simulink model "D53_LKAS_JLU_20200909_1512"  (R2018b)
settings: Solver=ode3  StartTime=0.0  StopTime=10.0  FixedStep=0.01  RelTol=1e-3  EnableMultiTasking=on
model workspace (MAT data in the model file):
  MCOS : class17 (value not decoded)
  MCOS : class17 (value not decoded)
  MCOS : class17 (value not decoded)
  MCOS : class17 (value not decoded)
  MCOS : class17 (value not decoded)
  MCOS : class17 (value not decoded)
  MCOS : class17 (value not decoded)
  MCOS : class17 (value not decoded)
  MCOS : class17 (value not decoded)
  MCOS : class17 (value not decoded)
  MCOS : class17 (value not decoded)
  MCOS : class17 (value not decoded)
  MCOS : class17 (value not decoded)
  MCOS : class17 (value not decoded)
  MCOS : class17 (value not decoded)
  MCOS : class17 (value not decoded)
  MCOS : class17 (value not decoded)
  MCOS : class17 (value not decoded)
  MCOS : class17 (value not decoded)
  MCOS : class17 (value not decoded)
  MCOS : class17 (value not decoded)
  MCOS : class17 (value not decoded)
  MCOS : class17 (value not decoded)
  MCOS : class17 (value not decoded)
  MCOS : class17 (value not decoded)
  MCOS : class17 (value not decoded)
  MCOS : class17 (value not decoded)
  MCOS : class17 (value not decoded)
  MCOS : class17 (value not decoded)
  MCOS : class17 (value not decoded)
  MCOS : class17 (value not decoded)
  MCOS : class17 (value not decoded)
  MCOS : class17 (value not decoded)
  MCOS : class17 (value not decoded)
  MCOS : class17 (value not decoded)
  MCOS : class17 (value not decoded)
  MCOS : class17 (value not decoded)
  MCOS : class17 (value not decoded)
  MCOS : class17 (value not decoded)
  MCOS : class17 (value not decoded)
  MCOS : class17 (value not decoded)
  MCOS : class17 (value not decoded)
  MCOS : class17 (value not decoded)
  MCOS : class17 (value not decoded)
  MCOS : class17 (value not decoded)
  MCOS : class17 (value not decoded)
  MCOS : class17 (value not decoded)
  MCOS : class17 (value not decoded)
  MCOS : class17 (value not decoded)
  MCOS : class17 (value not decoded)
  MCOS : class17 (value not decoded)
  MCOS : class17 (value not decoded)
  MCOS : class17 (value not decoded)
  MCOS : class17 (value not decoded)
  MCOS : class17 (value not decoded)
  MCOS : class17 (value not decoded)
  MCOS : class17 (value not decoded)
  MCOS : class17 (value not decoded)
  MCOS : class17 (value not decoded)
  MCOS : class17 (value not decoded)
  MCOS : class17 (value not decoded)
  MCOS : class17 (value not decoded)
  MCOS : class17 (value not decoded)
  MCOS : class17 (value not decoded)
  MCOS : class17 (value not decoded)
  MCOS : class17 (value not decoded)
  MCOS : class17 (value not decoded)
  MCOS : class17 (value not decoded)
  MCOS : class17 (value not decoded)
  MCOS : class17 (value not decoded)
  MCOS : class17 (value not decoded)
  MCOS : class17 (value not decoded)
  MCOS : class17 (value not decoded)
  MCOS : class17 (value not decoded)
  MCOS : class17 (value not decoded)
  MCOS : class17 (value not decoded)
  MCOS : class17 (value not decoded)
  MCOS : class17 (value not decoded)
  MCOS : class17 (value not decoded)
  MCOS : class17 (value not decoded)
  MCOS : class17 (value not decoded)
  MCOS : class17 (value not decoded)
  MCOS : class17 (value not decoded)
  MCOS : class17 (value not decoded)
  MCOS : class17 (value not decoded)
  MCOS : class17 (value not decoded)
  MCOS : class17 (value not decoded)
  MCOS : class17 (value not decoded)
  MCOS : class17 (value not decoded)
undefined symbols (not defined in the file): LKA_CarWidth, LKA_SampleTime, LKA_StrRatio_C, LKA_Veh2CamL_C, LKA_Veh2CamW_C, LKA_WhlBaseL_C, LL_CompSWA_C, LL_CrvtPrvwT_C, LL_DesDvt_C, LL_DvtComp_C, LL_DvtPrvwT_C, LL_DvtSpdDet_vDvtSpdMin_C, LL_HdAgExT_C, LL_HdAgPrvwT_C, LL_LAccMax_C, LL_LAccRMax_C, LL_LDW_EarliestWarnLine_C, LL_LDW_LatestWarnLine_C, LL_LDWS_SUPPRESS_HEADING, LL_LFClb_TFC_DiffCtlBalance, LL_LFClb_TFC_DiffCtrlMaxSWA, LL_LFClb_TFC_DiffCtrlRatio, LL_LFClb_TFC_facmGainLutGain1_C, LL_LFClb_TFC_facmGainLutGain2_C, LL_LFClb_TFC_facmIntegRatio, LL_LFClb_TFC_facmKlat_C, LL_LFClb_TFC_FfCtlRatio_C, LL_LFClb_TFC_phiIntegCtlMaxSWA_C, LL_LFClb_TFC_tiKlatPrvwT_C, LL_LFClb_TFC_vGainLutVehSpdLwr_C, LL_LFClb_TFC_vGainLutVehSpdUpr_C, LL_LKA_EarliestWarnLine_C, LL_LKA_LatestWarnLine_C, LL_LKAExPrcs_ExitC0Dvt, LL_LKAExPrcs_ExitC0Swt, LL_LKAExPrcs_tiExitTime1, LL_LKAExPrcs_tiExitTime2, LL_LKAExPrcs_tiExitTime3, LL_LKAS_OUT_OF_CONTROL_LAT_VEL, LL_LKAS_OUT_OF_CONTROL_TTLC, LL_LKASWASyn_M0, LL_LKASWASyn_M1, LL_LKASWASyn_M2, LL_LKASWASyn_M3K, LL_LKASWASyn_SWAaddMax, LL_LKASWASyn_T2, LL_LKASWASyn_tiTrqSwaRtTime, LL_LKASWASyn_tiTrqSwaTime, LL_LKASWASyn_TrqMax, LL_LKASWASyn_TrqSwaAddSwt, LL_LKASWASyn_TrqSwaRateDiff, LL_LSpdCompT_C, LL_lStpLngth_C, LL_MAX_DELAY_EPSSTAR_TIME, LL_MAX_DRIVER_TORQUE_DISABLE, LL_MAX_DRIVER_TORQUE_ENABLE, LL_MAX_LANE_WIDTH_DISABLE, LL_MAX_LANE_WIDTH_ENABLE, LL_MAX_LAT_ACC_DISABLE, LL_MAX_LAT_ACC_ENABLE ... (+30)
libraries: simulink x134, canmsglib x50, dspstat3 x3, simulink_extras x1
(part 4 of 17)

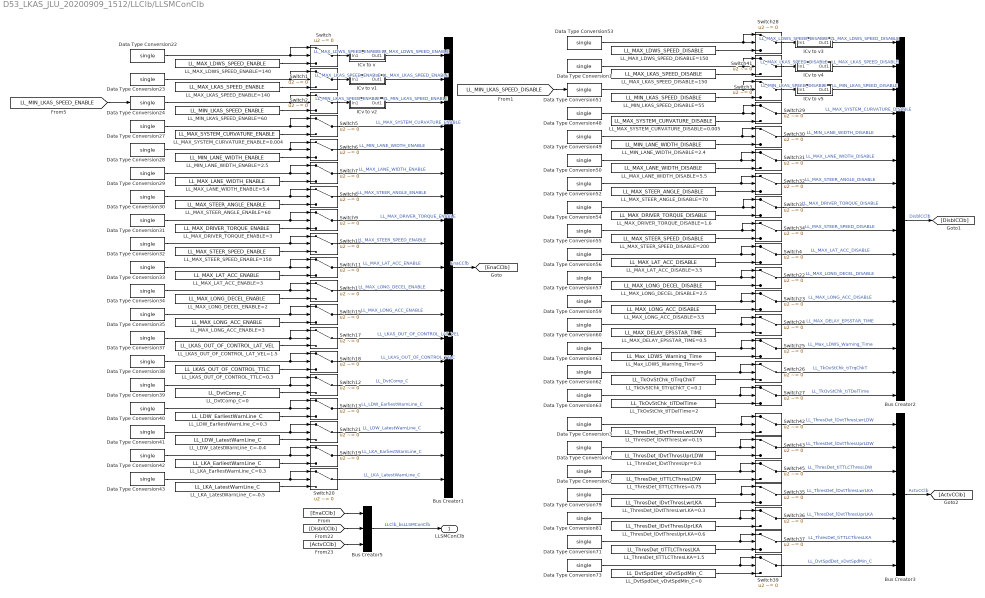
== system D53_LKAS_JLU_20200909_1512/LLClb/LLSMConClb ==
  Bus Creator1 : BusCreator  Inputs=19
  Bus Creator2 : BusCreator  Inputs=16
  Bus Creator3 : BusCreator  Inputs=7
  Bus Creator5 : BusCreator  Inputs=3
  Data Type Conversion{1..4,22..24,27..35,37..43,48..57,59..63,71,73,79,81} (42 alike) : DataTypeConversion  OutDataTypeStr=single
  ICv to v : Subsystem
  ICv to v1 : Subsystem
  ICv to v2 : Subsystem
  ICv to v3 : Subsystem
  ICv to v4 : Subsystem
  ICv to v5 : Subsystem
  LL_DvtComp_C=0 : Constant  Value=LL_DvtComp_C  OutDataTypeStr=single
  LL_DvtSpdDet_vDvtSpdMin_C=0 : Constant  Value=LL_DvtSpdDet_vDvtSpdMin_C  OutDataTypeStr=single
  LL_LDW_EarliestWarnLine_C=0.3 : Constant  Value=LL_LDW_EarliestWarnLine_C  OutDataTypeStr=single
  LL_LDW_LatestWarnLine_C=-0.4 : Constant  Value=LL_LDW_LatestWarnLine_C  OutDataTypeStr=single
  LL_LKAS_OUT_OF_CONTROL_LAT_VEL=1.5 : Constant  Value=LL_LKAS_OUT_OF_CONTROL_LAT_VEL  OutDataTypeStr=single
  LL_LKAS_OUT_OF_CONTROL_TTLC=0.3 : Constant  Value=LL_LKAS_OUT_OF_CONTROL_TTLC  OutDataTypeStr=single
  LL_LKA_EarliestWarnLine_C=0.3 : Constant  Value=LL_LKA_EarliestWarnLine_C  OutDataTypeStr=single
  LL_LKA_LatestWarnLine_C=-0.5 : Constant  Value=LL_LKA_LatestWarnLine_C  OutDataTypeStr=single
  LL_MAX_DELAY_EPSSTAR_TIME=0.5 : Constant  Value=LL_MAX_DELAY_EPSSTAR_TIME  OutDataTypeStr=single
  LL_MAX_DRIVER_TORQUE_DISABLE=1.6 : Constant  Value=LL_MAX_DRIVER_TORQUE_DISABLE  OutDataTypeStr=single
  LL_MAX_DRIVER_TORQUE_ENABLE=3 : Constant  Value=LL_MAX_DRIVER_TORQUE_ENABLE  OutDataTypeStr=single
  LL_MAX_LANE_WIDTH_DISABLE=5.5 : Constant  Value=LL_MAX_LANE_WIDTH_DISABLE  OutDataTypeStr=single
  LL_MAX_LANE_WIDTH_ENABLE=5.4 : Constant  Value=LL_MAX_LANE_WIDTH_ENABLE  OutDataTypeStr=single
  LL_MAX_LAT_ACC_DISABLE=3.5 : Constant  Value=LL_MAX_LAT_ACC_DISABLE  OutDataTypeStr=single
  LL_MAX_LAT_ACC_ENABLE=3 : Constant  Value=LL_MAX_LAT_ACC_ENABLE  OutDataTypeStr=single
  LL_MAX_LDWS_SPEED_DISABLE=150 : Constant  Value=LL_MAX_LDWS_SPEED_DISABLE  OutDataTypeStr=single
  LL_MAX_LDWS_SPEED_ENABLE=140 : Constant  Value=LL_MAX_LDWS_SPEED_ENABLE  OutDataTypeStr=single
  LL_MAX_LKAS_SPEED_DISABLE=150 : Constant  Value=LL_MAX_LKAS_SPEED_DISABLE  OutDataTypeStr=single
  LL_MAX_LKAS_SPEED_ENABLE=140 : Constant  Value=LL_MAX_LKAS_SPEED_ENABLE  OutDataTypeStr=single
  LL_MAX_LONG_ACC_DISABLE=3.5 : Constant  Value=LL_MAX_LONG_ACC_DISABLE  OutDataTypeStr=single
  LL_MAX_LONG_ACC_ENABLE=3 : Constant  Value=LL_MAX_LONG_ACC_ENABLE  OutDataTypeStr=single
  LL_MAX_LONG_DECEL_DISABLE=2.5 : Constant  Value=LL_MAX_LONG_DECEL_DISABLE  OutDataTypeStr=single
  LL_MAX_LONG_DECEL_ENABLE=2 : Constant  Value=LL_MAX_LONG_DECEL_ENABLE  OutDataTypeStr=single
  LL_MAX_STEER_ANGLE_DISABLE=70 : Constant  Value=LL_MAX_STEER_ANGLE_DISABLE  OutDataTypeStr=single
  LL_MAX_STEER_ANGLE_ENABLE=60 : Constant  Value=LL_MAX_STEER_ANGLE_ENABLE  OutDataTypeStr=single
  LL_MAX_STEER_SPEED_DISABLE=200 : Constant  Value=LL_MAX_STEER_SPEED_DISABLE  OutDataTypeStr=single
  LL_MAX_STEER_SPEED_ENABLE=150 : Constant  Value=LL_MAX_STEER_SPEED_ENABLE  OutDataTypeStr=single
  LL_MAX_SYSTEM_CURVATURE_DISABLE=0.005 : Constant  Value=LL_MAX_SYSTEM_CURVATURE_DISABLE  OutDataTypeStr=single
  LL_MAX_SYSTEM_CURVATURE_ENABLE=0.004 : Constant  Value=LL_MAX_SYSTEM_CURVATURE_ENABLE  OutDataTypeStr=single
  LL_MIN_LANE_WIDTH_DISABLE=2.4 : Constant  Value=LL_MIN_LANE_WIDTH_DISABLE  OutDataTypeStr=single
  LL_MIN_LANE_WIDTH_ENABLE=2.5 : Constant  Value=LL_MIN_LANE_WIDTH_ENABLE  OutDataTypeStr=single
  LL_MIN_LKAS_SPEED_DISABLE=55 : Constant  Value=LL_MIN_LKAS_SPEED_DISABLE  OutDataTypeStr=single
  LL_MIN_LKAS_SPEED_ENABLE=60 : Constant  Value=LL_MIN_LKAS_SPEED_ENABLE  OutDataTypeStr=single
  LL_Max_LDWS_Warning_Time=5 : Constant  Value=LL_Max_LDWS_Warning_Time  OutDataTypeStr=single
  LL_ThresDet_lDvtThresLwr=0.15 : Constant  Value=LL_ThresDet_lDvtThresLwrLDW  OutDataTypeStr=single
  LL_ThresDet_lDvtThresLwrLKA=0.3 : Constant  Value=LL_ThresDet_lDvtThresLwrLKA  OutDataTypeStr=single
  LL_ThresDet_lDvtThresUpr=0.3 : Constant  Value=LL_ThresDet_lDvtThresUprLDW  OutDataTypeStr=single
  LL_ThresDet_lDvtThresUprLKA=0.6 : Constant  Value=LL_ThresDet_lDvtThresUprLKA  OutDataTypeStr=single
  LL_ThresDet_tiTTLCThres=0.75 : Constant  Value=LL_ThresDet_tiTTLCThresLDW  OutDataTypeStr=single
  LL_ThresDet_tiTTLCThresLKA=1.5 : Constant  Value=LL_ThresDet_tiTTLCThresLKA  OutDataTypeStr=single
  LL_TkOvStChk_tiTDelTime=2 : Constant  Value=LL_TkOvStChk_tiTDelTime  OutDataTypeStr=single
  LL_TkOvStChk_tiTrqChkT_C=0.1 : Constant  Value=LL_TkOvStChk_tiTrqChkT  OutDataTypeStr=single
  Switch{,1..15,17..37,39,41..43,45} (42 alike) : Switch  Criteria=u2 ~= 0  OutDataTypeStr=single
  LLSMConClb : Outport
  wires:
  Data Type Conversion39/1 -> Switch12/2, Switch12/1
  Switch10/1 -> Bus Creator1/9  "LL_MAX_STEER_SPEED_ENABLE"
  LL_MAX_LANE_WIDTH_ENABLE=5.4/1 -> Switch7/3
  Data Type Conversion42/1 -> Switch19/2, Switch19/1
  ICv to v2/1(Out1) -> Bus Creator1/3  "LL_MIN_LKAS_SPEED_ENABLE"
  LL_LKA_LatestWarnLine_C=-0.5/1 -> Switch20/3
  Data Type Conversion40/1 -> Switch13/2, Switch13/1
  LL_MAX_STEER_ANGLE_ENABLE=60/1 -> Switch8/3
  Data Type Conversion38/1 -> Switch18/2, Switch18/1
  Data Type Conversion43/1 -> Switch20/2, Switch20/1
  LL_MIN_LANE_WIDTH_ENABLE=2.5/1 -> Switch6/3
  Switch6/1 -> Bus Creator1/5  "LL_MIN_LANE_WIDTH_ENABLE"
  Switch17/1 -> Bus Creator1/13  "LL_LKAS_OUT_OF_CONTROL_LAT_VEL"
  LL_MAX_LONG_DECEL_ENABLE=2/1 -> Switch14/3
  Data Type Conversion30/1 -> Switch8/2, Switch8/1
  Data Type Conversion27/1 -> Switch5/2, Switch5/1
  Data Type Conversion31/1 -> Switch9/2, Switch9/1
  Data Type Conversion28/1 -> Switch6/2, Switch6/1
  LL_LKAS_OUT_OF_CONTROL_LAT_VEL=1.5/1 -> Switch17/3
  Data Type Conversion23/1 -> Switch1/2, Switch1/1
  LL_MIN_LKAS_SPEED_ENABLE=60/1 -> Switch2/3
  Data Type Conversion22/1 -> Switch/2, Switch/1
  Data Type Conversion24/1 -> Switch2/2, Switch2/1
  LL_MAX_LAT_ACC_ENABLE=3/1 -> Switch11/3
  LL_MAX_LDWS_SPEED_ENABLE=140/1 -> Switch/3
  Switch12/1 -> Bus Creator1/15  "LL_DvtComp_C"
  LL_LDW_LatestWarnLine_C=-0.4/1 -> Switch21/3
  Data Type Conversion29/1 -> Switch7/2, Switch7/1
  LL_MAX_LONG_ACC_ENABLE=3/1 -> Switch15/3
  LL_MAX_DRIVER_TORQUE_ENABLE=3/1 -> Switch9/3
  Data Type Conversion35/1 -> Switch15/2, Switch15/1
  LL_DvtComp_C=0/1 -> Switch12/3
  Switch19/1 -> Bus Creator1/18  "LL_LKA_EarliestWarnLine_C"
  LL_LKAS_OUT_OF_CONTROL_TTLC=0.3/1 -> Switch18/3
  Data Type Conversion32/1 -> Switch10/2, Switch10/1
  Data Type Conversion37/1 -> Switch17/2, Switch17/1
  Data Type Conversion33/1 -> Switch11/2, Switch11/1
  Switch7/1 -> Bus Creator1/6  "LL_MAX_LANE_WIDTH_ENABLE"
  Data Type Conversion34/1 -> Switch14/2, Switch14/1
  LL_LKA_EarliestWarnLine_C=0.3/1 -> Switch19/3
  Switch15/1 -> Bus Creator1/12  "LL_MAX_LONG_ACC_ENABLE"
  Switch18/1 -> Bus Creator1/14  "LL_LKAS_OUT_OF_CONTROL_TTLC"
  Switch21/1 -> Bus Creator1/17  "LL_LDW_LatestWarnLine_C"
  ICv to v/1(Out1) -> Bus Creator1/1  "LL_MAX_LDWS_SPEED_ENABLE"
  Switch20/1 -> Bus Creator1/19  "LL_LKA_LatestWarnLine_C"
  Switch14/1 -> Bus Creator1/11  "LL_MAX_LONG_DECEL_ENABLE"
  Switch13/1 -> Bus Creator1/16  "LL_LDW_EarliestWarnLine_C"
  Switch9/1 -> Bus Creator1/8  "LL_MAX_DRIVER_TORQUE_ENABLE"
  LL_MAX_STEER_SPEED_ENABLE=150/1 -> Switch10/3
  LL_MAX_SYSTEM_CURVATURE_ENABLE=0.004/1 -> Switch5/3
  Switch5/1 -> Bus Creator1/4  "LL_MAX_SYSTEM_CURVATURE_ENABLE"
  Switch8/1 -> Bus Creator1/7  "LL_MAX_STEER_ANGLE_ENABLE"
  Data Type Conversion41/1 -> Switch21/2, Switch21/1
  LL_LDW_EarliestWarnLine_C=0.3/1 -> Switch13/3
  ICv to v1/1(Out1) -> Bus Creator1/2  "LL_MAX_LKAS_SPEED_ENABLE"
  LL_MAX_LKAS_SPEED_ENABLE=140/1 -> Switch1/3
  Switch11/1 -> Bus Creator1/10  "LL_MAX_LAT_ACC_ENABLE"
  Data Type Conversion54/1 -> Switch33/2, Switch33/1
  Data Type Conversion63/1 -> Switch27/2, Switch27/1
  Data Type Conversion52/1 -> Switch32/2, Switch32/1
  Data Type Conversion61/1 -> Switch25/2, Switch25/1
  Switch26/1 -> Bus Creator2/15  "LL_TkOvStChk_tiTrqChkT"
  LL_MIN_LKAS_SPEED_DISABLE=55/1 -> Switch3/3
  Data Type Conversion60/1 -> Switch24/2, Switch24/1
  Data Type Conversion59/1 -> Switch23/2, Switch23/1
  Data Type Conversion49/1 -> Switch30/2, Switch30/1
  Switch30/1 -> Bus Creator2/5  "LL_MIN_LANE_WIDTH_DISABLE"
  Data Type Conversion62/1 -> Switch26/2, Switch26/1
  LL_MAX_LONG_DECEL_DISABLE=2.5/1 -> Switch22/3
  Switch25/1 -> Bus Creator2/14  "LL_Max_LDWS_Warning_Time"
  Data Type Conversion57/1 -> Switch22/1, Switch22/2
  Switch29/1 -> Bus Creator2/4  "LL_MAX_SYSTEM_CURVATURE_DISABLE"
  Data Type Conversion48/1 -> Switch29/2, Switch29/1
  LL_MAX_SYSTEM_CURVATURE_DISABLE=0.005/1 -> Switch29/3
  Switch23/1 -> Bus Creator2/12  "LL_MAX_LONG_ACC_DISABLE"
  LL_MAX_DELAY_EPSSTAR_TIME=0.5/1 -> Switch24/3
  Data Type Conversion53/1 -> Switch28/2, Switch28/1
  LL_MAX_DRIVER_TORQUE_DISABLE=1.6/1 -> Switch33/3
  LL_MAX_LANE_WIDTH_DISABLE=5.5/1 -> Switch31/3
  LL_TkOvStChk_tiTrqChkT_C=0.1/1 -> Switch26/3
  LL_MAX_LDWS_SPEED_DISABLE=150/1 -> Switch28/3
  Switch4/1 -> Bus Creator2/10  "LL_MAX_LAT_ACC_DISABLE"
  Data Type Conversion50/1 -> Switch31/2, Switch31/1
  Data Type Conversion51/1 -> Switch3/1, Switch3/2
  LL_MAX_LAT_ACC_DISABLE=3.5/1 -> Switch4/3
  Data Type Conversion55/1 -> Switch34/2, Switch34/1
  Switch33/1 -> Bus Creator2/8  "LL_MAX_DRIVER_TORQUE_DISABLE"
  LL_MIN_LANE_WIDTH_DISABLE=2.4/1 -> Switch30/3
  LL_Max_LDWS_Warning_Time=5/1 -> Switch25/3
  LL_MAX_STEER_SPEED_DISABLE=200/1 -> Switch34/3
  LL_MAX_LONG_ACC_DISABLE=3.5/1 -> Switch23/3
  Switch22/1 -> Bus Creator2/11  "LL_MAX_LONG_DECEL_DISABLE"
  Switch24/1 -> Bus Creator2/13  "LL_MAX_DELAY_EPSSTAR_TIME"
  Switch32/1 -> Bus Creator2/7  "LL_MAX_STEER_ANGLE_DISABLE"
  Switch34/1 -> Bus Creator2/9  "LL_MAX_STEER_SPEED_DISABLE"
  Switch31/1 -> Bus Creator2/6  "LL_MAX_LANE_WIDTH_DISABLE"
  Data Type Conversion56/1 -> Switch4/1, Switch4/2
  LL_MAX_STEER_ANGLE_DISABLE=70/1 -> Switch32/3
  ICv to v5/1(Out1) -> Bus Creator2/3  "LL_MIN_LKAS_SPEED_DISABLE"
  LL_TkOvStChk_tiTDelTime=2/1 -> Switch27/3
  Switch27/1 -> Bus Creator2/16  "LL_TkOvStChk_tiTDelTime"
  Bus Creator2/1 -> [DisblCClb]  "DisblCClb"
  Data Type Conversion81/1 -> Switch36/2, Switch36/1
  LL_ThresDet_tiTTLCThresLKA=1.5/1 -> Switch37/3
  LL_DvtSpdDet_vDvtSpdMin_C=0/1 -> Switch39/3
  Data Type Conversion71/1 -> Switch37/2, Switch37/1
  LL_ThresDet_lDvtThresLwrLKA=0.3/1 -> Switch35/3
  Data Type Conversion79/1 -> Switch35/1, Switch35/2
  LL_ThresDet_lDvtThresUprLKA=0.6/1 -> Switch36/3
  Switch39/1 -> Bus Creator3/7  "LL_DvtSpdDet_vDvtSpdMin_C"
  Switch37/1 -> Bus Creator3/6  "LL_ThresDet_tiTTLCThresLKA"
  Switch35/1 -> Bus Creator3/4  "LL_ThresDet_lDvtThresLwrLKA"
  Switch36/1 -> Bus Creator3/5  "LL_ThresDet_lDvtThresUprLKA"
  Data Type Conversion73/1 -> Switch39/1, Switch39/2
  Bus Creator1/1 -> [EnaCClb]  "EnaCClb"
  Bus Creator3/1 -> [ActvCClb]  "ActvCClb"
  [EnaCClb] -> Bus Creator5/1
  [DisblCClb] -> Bus Creator5/2
  [ActvCClb] -> Bus Creator5/3
  Bus Creator5/1 -> LLSMConClb/1  "LLClb_bsLLSMConClb"
  ICv to v4/1(Out1) -> Bus Creator2/2  "LL_MAX_LKAS_SPEED_DISABLE"
  Data Type Conversion1/1 -> Switch41/2, Switch41/1
  LL_MAX_LKAS_SPEED_DISABLE=150/1 -> Switch41/3
  Switch43/1 -> Bus Creator3/2  "LL_ThresDet_lDvtThresUprLDW"
  Switch42/1 -> Bus Creator3/1  "LL_ThresDet_lDvtThresLwrLDW"
  Switch45/1 -> Bus Creator3/3  "LL_ThresDet_tiTTLCThresLDW"
  LL_ThresDet_lDvtThresUpr=0.3/1 -> Switch43/3
  Data Type Conversion3/1 -> Switch42/2, Switch42/1
  LL_ThresDet_lDvtThresLwr=0.15/1 -> Switch42/3
  Data Type Conversion2/1 -> Switch45/1, Switch45/2
  LL_ThresDet_tiTTLCThres=0.75/1 -> Switch45/3
  Data Type Conversion4/1 -> Switch43/1, Switch43/2
  Switch/1 -> ICv to v/1(In1)  "LL_MAX_LDWS_SPEED_ENABLE"
  Switch1/1 -> ICv to v1/1(In1)  "LL_MAX_LKAS_SPEED_ENABLE"
  Switch2/1 -> ICv to v2/1(In1)  "LL_MIN_LKAS_SPEED_ENABLE"
  Switch28/1 -> ICv to v3/1(In1)  "LL_MAX_LDWS_SPEED_DISABLE"
  ICv to v3/1(Out1) -> Bus Creator2/1  "LL_MAX_LDWS_SPEED_DISABLE"
  Switch41/1 -> ICv to v4/1(In1)  "LL_MAX_LKAS_SPEED_DISABLE"
  Switch3/1 -> ICv to v5/1(In1)  "LL_MIN_LKAS_SPEED_DISABLE"
  [LL_MIN_LKAS_SPEED_ENABLE] -> Data Type Conversion24/1
  [LL_MIN_LKAS_SPEED_DISABLE] -> Data Type Conversion51/1

== system D53_LKAS_JLU_20200909_1512/LLOut/D53_EPS_Control_LKA ==
  LKA_STATE_in : Inport
  LXA_ACTIVATION_in : Inport  Port=2
  LKA_TRQ_FACT_REQ_in : Inport  Port=3
  COLUMN_ANGLE_SETPOINT_in : Inport  Port=4
  Constant{2..9} (8 alike) : Constant  Value=0  OutDataTypeStr=single
  Data Type Conversion : DataTypeConversion  OutDataTypeStr=single
  DMD_DELEST_ABS_ESP : Outport
  REQ_DECON_ASR : Outport  Port=2
  LKA_TRQ_FACT_REQ : Outport  Port=3
  COLUMN_ANGLE_SETPOINT : Outport  Port=4
  ACPK_VAL_REQUEST_BSI : Outport  Port=5
  DMD_DELEST_EASYMOVE : Outport  Port=6
  LKA_STATE : Outport  Port=7
  LXA_ACTIVATION : Outport  Port=8
  DMD_DELEST_DA : Outport  Port=9
  TRAILER_DETECTION : Outport  Port=10
  CPT_PROCESS : Outport  Port=11
  CHKSUM_TRME : Outport  Port=12
  wires:
  LKA_STATE_in/1 -> Data Type Conversion/1
  Data Type Conversion/1 -> LKA_STATE/1
  COLUMN_ANGLE_SETPOINT_in/1 -> COLUMN_ANGLE_SETPOINT/1
  Constant2/1 -> DMD_DELEST_DA/1
  LXA_ACTIVATION_in/1 -> LXA_ACTIVATION/1
  LKA_TRQ_FACT_REQ_in/1 -> LKA_TRQ_FACT_REQ/1
  Constant3/1 -> TRAILER_DETECTION/1
  Constant4/1 -> DMD_DELEST_EASYMOVE/1
  Constant5/1 -> DMD_DELEST_ABS_ESP/1
  Constant6/1 -> CHKSUM_TRME/1
  Constant7/1 -> CPT_PROCESS/1
  Constant8/1 -> REQ_DECON_ASR/1
  Constant9/1 -> ACPK_VAL_REQUEST_BSI/1

== system D53_LKAS_JLU_20200909_1512/LLOut/D53_EPS_Control_LKA1 ==
  LKA_STATE_in : Inport
  LXA_ACTIVATION_in : Inport  Port=2
  LKA_TRQ_FACT_REQ_in : Inport  Port=3
  COLUMN_ANGLE_SETPOINT_in : Inport  Port=4
  Constant{2..9} (8 alike) : Constant  Value=0  OutDataTypeStr=single
  Data Type Conversion : DataTypeConversion  OutDataTypeStr=single
  DMD_DELEST_ABS_ESP : Outport
  REQ_DECON_ASR : Outport  Port=2
  LKA_TRQ_FACT_REQ : Outport  Port=3
  COLUMN_ANGLE_SETPOINT : Outport  Port=4
  ACPK_VAL_REQUEST_BSI : Outport  Port=5
  DMD_DELEST_EASYMOVE : Outport  Port=6
  LKA_STATE : Outport  Port=7
  LXA_ACTIVATION : Outport  Port=8
  DMD_DELEST_DA : Outport  Port=9
  TRAILER_DETECTION : Outport  Port=10
  CPT_PROCESS : Outport  Port=11
  CHKSUM_TRME : Outport  Port=12
  wires:
  Constant9/1 -> ACPK_VAL_REQUEST_BSI/1
  Constant8/1 -> REQ_DECON_ASR/1
  Constant7/1 -> CPT_PROCESS/1
  Constant6/1 -> CHKSUM_TRME/1
  Constant5/1 -> DMD_DELEST_ABS_ESP/1
  Constant4/1 -> DMD_DELEST_EASYMOVE/1
  Constant3/1 -> TRAILER_DETECTION/1
  LKA_TRQ_FACT_REQ_in/1 -> LKA_TRQ_FACT_REQ/1
  LXA_ACTIVATION_in/1 -> LXA_ACTIVATION/1
  Constant2/1 -> DMD_DELEST_DA/1
  COLUMN_ANGLE_SETPOINT_in/1 -> COLUMN_ANGLE_SETPOINT/1
  Data Type Conversion/1 -> LKA_STATE/1
  LKA_STATE_in/1 -> Data Type Conversion/1

== system D53_LKAS_JLU_20200909_1512/LLOut/D53_HMI_Control_LKA ==
  LL_bsLLHMI : Inport
  Bus Selector3 : BusSelector  OutputSignals=Hands_off_warning,HMI_Popup_Status,LDW_Flag,LDW_Status_Display,LKA_action_indication,LKA_Status_Display,Vehicle_Lane_Display
  Constant{,1..7} (8 alike) : Constant  Value=0  OutDataTypeStr=uint16
  ECU_operating_phase : Outport
  HMI_Popup_Status : Outport  Port=2
  Hands_off_warning : Outport  Port=3
  ISA_Popup_text : Outport  Port=4
  ISA_Sign_Type : Outport  Port=5
  ISA_Status : Outport  Port=6
  ISA_Value : Outport  Port=7
  LDW_Flag : Outport  Port=8
  LDW_Status_Display : Outport  Port=9
  LKA_Mode_from_Camera : Outport  Port=10
  LKA_Status_Display : Outport  Port=11
  LKA_Switch_State : Outport  Port=12
  LKA_action_indication : Outport  Port=13
  TSR_Vision_Only_Sign_Type : Outport  Port=14
  Vehicle_Lane_Display : Outport  Port=15
  wires:
  Bus Selector3/1 -> Hands_off_warning/1  "<Hands_off_warning>"
  Bus Selector3/3 -> LDW_Flag/1  "<LDW_Flag>"
  Bus Selector3/4 -> LDW_Status_Display/1  "<LDW_Status_Display>"
  Bus Selector3/5 -> LKA_action_indication/1  "<LKA_action_indication>"
  Bus Selector3/6 -> LKA_Status_Display/1  "<LKA_Status_Display>"
  Bus Selector3/7 -> Vehicle_Lane_Display/1  "<Vehicle_Lane_Display>"
  Bus Selector3/2 -> HMI_Popup_Status/1  "<HMI_Popup_Status>"
  LL_bsLLHMI/1 -> Bus Selector3/1
  Constant/1 -> ECU_operating_phase/1
  Constant1/1 -> ISA_Popup_text/1
  Constant2/1 -> ISA_Sign_Type/1
  Constant4/1 -> ISA_Value/1
  Constant3/1 -> ISA_Status/1
  Constant5/1 -> LKA_Mode_from_Camera/1
  Constant6/1 -> LKA_Switch_State/1
  Constant7/1 -> TSR_Vision_Only_Sign_Type/1

== system D53_LKAS_JLU_20200909_1512/LLOut/D53_HMI_Control_LKA1 ==
  LL_bsLLHMI : Inport
  Bus Selector3 : BusSelector  OutputSignals=Hands_off_warning,HMI_Popup_Status,LDW_Flag,LDW_Status_Display,LKA_action_indication,LKA_Status_Display,Vehicle_Lane_Display
  Constant{,1..7} (8 alike) : Constant  Value=0  OutDataTypeStr=uint16
  ECU_operating_phase : Outport
  HMI_Popup_Status : Outport  Port=2
  Hands_off_warning : Outport  Port=3
  ISA_Popup_text : Outport  Port=4
  ISA_Sign_Type : Outport  Port=5
  ISA_Status : Outport  Port=6
  ISA_Value : Outport  Port=7
  LDW_Flag : Outport  Port=8
  LDW_Status_Display : Outport  Port=9
  LKA_Mode_from_Camera : Outport  Port=10
  LKA_Status_Display : Outport  Port=11
  LKA_Switch_State : Outport  Port=12
  LKA_action_indication : Outport  Port=13
  TSR_Vision_Only_Sign_Type : Outport  Port=14
  Vehicle_Lane_Display : Outport  Port=15
  wires:
  Constant7/1 -> TSR_Vision_Only_Sign_Type/1
  Constant6/1 -> LKA_Switch_State/1
  Constant5/1 -> LKA_Mode_from_Camera/1
  Constant3/1 -> ISA_Status/1
  Constant4/1 -> ISA_Value/1
  Constant2/1 -> ISA_Sign_Type/1
  Constant1/1 -> ISA_Popup_text/1
  Constant/1 -> ECU_operating_phase/1
  LL_bsLLHMI/1 -> Bus Selector3/1
  Bus Selector3/2 -> HMI_Popup_Status/1  "<HMI_Popup_Status>"
  Bus Selector3/7 -> Vehicle_Lane_Display/1  "<Vehicle_Lane_Display>"
  Bus Selector3/6 -> LKA_Status_Display/1  "<LKA_Status_Display>"
  Bus Selector3/5 -> LKA_action_indication/1  "<LKA_action_indication>"
  Bus Selector3/4 -> LDW_Status_Display/1  "<LDW_Status_Display>"
  Bus Selector3/3 -> LDW_Flag/1  "<LDW_Flag>"
  Bus Selector3/1 -> Hands_off_warning/1  "<Hands_off_warning>"

== system D53_LKAS_JLU_20200909_1512/Resource Initialization/CAN Setup ==
  S-Function : S-Function  FunctionName=CAN_Init_D  Parameters=uint8(Device_Index-1),uint8(CAN0_En),uint8(CAN0_Baudrate-1),uint8(CAN1_En),uint8(CAN1_Baudrate-1),uint8(CAN2_En),uint8(CAN2_Baudrate-1),uint8(CAN3_En),uint8(CAN3_Baudrate-1)  SFunctionDeploymentMode=off  EnableBusSupport=off

== system D53_LKAS_JLU_20200909_1512/Resource Initialization/DI ==

== system D53_LKAS_JLU_20200909_1512/Resource Initialization/DO ==

== system D53_LKAS_JLU_20200909_1512/Resource Initialization/SPI ==

== system D53_LKAS_JLU_20200909_1512/SignalBusCreator/DTC_Indicator ==
  Bus Creator11 : BusCreator  Inputs=2
  Constant{,2..21} (21 alike) : Constant  Value=0  OutDataTypeStr=uint8
  Mux : Mux  Inputs=16
  Mux1 : Mux  Inputs=5
  bsDTC_Indicator : Outport
  wires:
  Bus Creator11/1 -> bsDTC_Indicator/1  "bsDTC_Indicator"
  Mux/1 -> Bus Creator11/1  "LKAS_BSWDTC_Status"
  Constant/1 -> Mux/1  "CANEve_e_BusOff_PSA1CAN"
  Constant2/1 -> Mux/2  "CANEve_e_BusOff_SensorCAN"
  Constant4/1 -> Mux/4  "CANEve_e_Node_ESC_Validity"
  Constant3/1 -> Mux/3  "CANEve_e_Mute_PSA1CAN"
  Constant7/1 -> Mux/7  "CANEve_e_Node_TCU_Validity"
  Constant8/1 -> Mux/8  "CANEve_e_Node_GW_Validity"
  Constant6/1 -> Mux/6  "CANEve_e_Node_EMS_Validity"
  Constant5/1 -> Mux/5  "CANEve_e_Node_EPS_Validity"
  Constant13/1 -> Mux/13  "Reserved3"
  Constant14/1 -> Mux/14  "Reserved4"
  Constant16/1 -> Mux/16  "Reserved6"
  Constant15/1 -> Mux/15  "Reserved5"
  Constant11/1 -> Mux/11  "Reserved1"
  Constant12/1 -> Mux/12  "Reserved2"
  Constant10/1 -> Mux/10  "CANEve_e_Node_Camera_Validity"
  Constant9/1 -> Mux/9  "CANEve_e_Node_Radar_Validity"
  Constant17/1 -> Mux1/1  "ACC"
  Constant18/1 -> Mux1/2  "AEB"
  Constant19/1 -> Mux1/3  "LKA"
  Constant20/1 -> Mux1/4  "LDW"
  Constant21/1 -> Mux1/5  "TJA"
  Mux1/1 -> Bus Creator11/2  "Indicator_Status"

== system D53_LKAS_JLU_20200909_1512/SignalBusCreator/Fusion_AdditionalInf ==
  Bus Creator11 : BusCreator  Inputs=10
  Constant{,1..9} (10 alike) : Constant  Value=0  OutDataTypeStr=uint8
  Fusion_AdditionalInf : Outport
  wires:
  Constant1/1 -> Bus Creator11/2  "Radar_State"
  Constant3/1 -> Bus Creator11/4  "fusion_status"
  Constant6/1 -> Bus Creator11/7  "CONSTRUCTION_AREA"
  Constant2/1 -> Bus Creator11/3  "sensor_status"
  Constant4/1 -> Bus Creator11/5  "fusion_time_stamp"
  Constant5/1 -> Bus Creator11/6  "LANE_DETECT_ACTIV"
  Constant/1 -> Bus Creator11/1  "Carema_Status"
  Constant9/1 -> Bus Creator11/10  "SIGN_TSR_Sign_Type"
  Constant7/1 -> Bus Creator11/8  "ROAD_TYPE"
  Constant8/1 -> Bus Creator11/9  "SIGN_ISA_Value"
  Bus Creator11/1 -> Fusion_AdditionalInf/1  "Fusion_AdditionalInf"

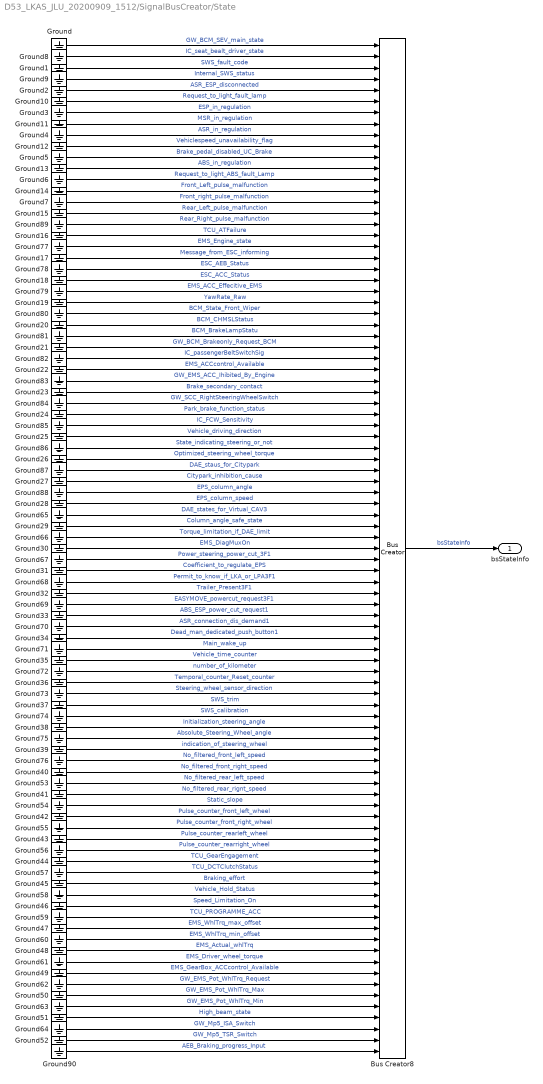
== system D53_LKAS_JLU_20200909_1512/SignalBusCreator/State ==
  Bus Creator8 : BusCreator  Inputs=91
  Ground{,1..90} (91 alike) : Ground
  bsStateInfo : Outport
  wires:
  Ground14/1 -> Bus Creator8/14  "Front_Left_pulse_malfunction"
  Ground8/1 -> Bus Creator8/2  "IC_seat_bealt_driver_state"
  Ground/1 -> Bus Creator8/1  "GW_BCM_SEV_main_state"
  Ground42/1 -> Bus Creator8/70  "Pulse_counter_front_left_wheel"
  Ground43/1 -> Bus Creator8/72  "Pulse_counter_rearleft_wheel"
  Ground12/1 -> Bus Creator8/10  "Vehiclespeed_unavailability_flag"
  Ground75/1 -> Bus Creator8/63  "Absolute_Steering_Wheel_angle"
  Ground71/1 -> Bus Creator8/55  "Main_wake_up"
  Ground44/1 -> Bus Creator8/74  "TCU_GearEngagement"
  Ground55/1 -> Bus Creator8/71  "Pulse_counter_front_right_wheel"
  Ground7/1 -> Bus Creator8/15  "Front_right_pulse_malfunction"
  Ground28/1 -> Bus Creator8/42  "EPS_column_speed"
  Ground79/1 -> Bus Creator8/23  "EMS_ACC_Effecitive_EMS"
  Ground77/1 -> Bus Creator8/19  "EMS_Engine_state"
  Ground80/1 -> Bus Creator8/25  "BCM_State_Front_Wiper"
  Ground41/1 -> Bus Creator8/68  "No_filtered_rear_rignt_speed"
  Ground67/1 -> Bus Creator8/47  "Power_steering_power_cut_3F1"
  Bus Creator8/1 -> bsStateInfo/1  "bsStateInfo"
  Ground90/1 -> Bus Creator8/91  "AEB_Braking_progress_Input"
  Ground38/1 -> Bus Creator8/62  "Initialization_steering_angle"
  Ground19/1 -> Bus Creator8/24  "YawRate_Raw"
  Ground83/1 -> Bus Creator8/31  "GW_EMS_ACC_Ihibited_By_Engine"
  Ground46/1 -> Bus Creator8/78  "Speed_Limitation_On"
  Ground51/1 -> Bus Creator8/88  "High_beam_state"
  Ground40/1 -> Bus Creator8/66  "No_filtered_front_right_speed"
  Ground3/1 -> Bus Creator8/7  "ESP_in_regulation"
  Ground36/1 -> Bus Creator8/58  "Temporal_counter_Reset_counter"
  Ground11/1 -> Bus Creator8/8  "MSR_in_regulation"
  Ground50/1 -> Bus Creator8/86  "GW_EMS_Pot_WhlTrq_Max"
  Ground10/1 -> Bus Creator8/6  "Request_to_light_fault_lamp"
  Ground13/1 -> Bus Creator8/12  "ABS_in_regulation"
  Ground5/1 -> Bus Creator8/11  "Brake_pedal_disabled_UC_Brake"
  Ground23/1 -> Bus Creator8/32  "Brake_secondary_contact"
  Ground60/1 -> Bus Creator8/81  "EMS_WhlTrq_min_offset"
  Ground15/1 -> Bus Creator8/16  "Rear_Left_pulse_malfunction"
  Ground24/1 -> Bus Creator8/34  "Park_brake_function_status"
  Ground6/1 -> Bus Creator8/13  "Request_to_light_ABS_fault_Lamp"
  Ground66/1 -> Bus Creator8/45  "Torque_limitation_if_DAE_limit"
  Ground72/1 -> Bus Creator8/57  "number_of_kilometer"
  Ground9/1 -> Bus Creator8/4  "Internal_SWS_status"
  Ground31/1 -> Bus Creator8/48  "Coefficient_to_regulate_EPS"
  Ground89/1 -> Bus Creator8/17  "Rear_Right_pulse_malfunction"
  Ground22/1 -> Bus Creator8/30  "EMS_ACCcontrol_Available"
  Ground73/1 -> Bus Creator8/59  "Steering_wheel_sensor_direction"
  Ground52/1 -> Bus Creator8/90  "GW_Mp5_TSR_Switch"
  Ground54/1 -> Bus Creator8/69  "Static_slope"
  Ground63/1 -> Bus Creator8/87  "GW_EMS_Pot_WhlTrq_Min"
  Ground25/1 -> Bus Creator8/36  "Vehicle_driving_direction"
  Ground69/1 -> Bus Creator8/51  "EASYMOVE_powercut_request3F1"
  Ground39/1 -> Bus Creator8/64  "indication_of_steering_wheel"
  Ground20/1 -> Bus Creator8/26  "BCM_CHMSLStatus"
  Ground57/1 -> Bus Creator8/75  "TCU_DCTClutchStatus"
  Ground27/1 -> Bus Creator8/40  "Citypark_inhibition_cause"
  Ground18/1 -> Bus Creator8/22  "ESC_ACC_Status"
  Ground65/1 -> Bus Creator8/43  "DAE_states_for_Virtual_CAV3"
  Ground84/1 -> Bus Creator8/33  "GW_SCC_RightSteeringWheelSwitch"
  Ground26/1 -> Bus Creator8/38  "Optimized_steering_wheel_torque"
  Ground33/1 -> Bus Creator8/52  "ABS_ESP_power_cut_request1"
  Ground17/1 -> Bus Creator8/20  "Message_from_ESC_informing"
  Ground29/1 -> Bus Creator8/44  "Column_angle_safe_state"
  Ground30/1 -> Bus Creator8/46  "EMS_DiagMuxOn"
  Ground68/1 -> Bus Creator8/49  "Permit_to_know_if_LKA_or_LPA3F1"
  Ground70/1 -> Bus Creator8/53  "ASR_connection_dis_demand1"
  Ground74/1 -> Bus Creator8/61  "SWS_calibration"
  Ground4/1 -> Bus Creator8/9  "ASR_in_regulation"
  Ground37/1 -> Bus Creator8/60  "SWS_trim"
  Ground53/1 -> Bus Creator8/67  "No_filtered_rear_left_speed"
  Ground2/1 -> Bus Creator8/5  "ASR_ESP_disconnected"
  Ground56/1 -> Bus Creator8/73  "Pulse_counter_rearright_wheel"
  Ground21/1 -> Bus Creator8/28  "GW_BCM_Brakeonly_Request_BCM"
  Ground59/1 -> Bus Creator8/79  "TCU_PROGRAMME_ACC"
  Ground47/1 -> Bus Creator8/80  "EMS_WhlTrq_max_offset"
  Ground45/1 -> Bus Creator8/76  "Braking_effort"
  Ground48/1 -> Bus Creator8/82  "EMS_Actual_whlTrq"
  Ground49/1 -> Bus Creator8/84  "EMS_GearBox_ACCcontrol_Available"
  Ground87/1 -> Bus Creator8/39  "DAE_staus_for_Citypark"
  Ground86/1 -> Bus Creator8/37  "State_indicating_steering_or_not"
  Ground85/1 -> Bus Creator8/35  "IC_FCW_Sensitivity"
  Ground78/1 -> Bus Creator8/21  "ESC_AEB_Status"
  Ground82/1 -> Bus Creator8/29  "IC_passengerBeltSwitchSig"
  Ground81/1 -> Bus Creator8/27  "BCM_BrakeLampStatu"
  Ground58/1 -> Bus Creator8/77  "Vehicle_Hold_Status"
  Ground64/1 -> Bus Creator8/89  "GW_Mp5_ISA_Switch"
  Ground35/1 -> Bus Creator8/56  "Vehicle_time_counter"
  Ground34/1 -> Bus Creator8/54  "Dead_man_dedicated_push_button1"
  Ground32/1 -> Bus Creator8/50  "Trailer_Present3F1"
  Ground61/1 -> Bus Creator8/83  "EMS_Driver_wheel_torque"
  Ground76/1 -> Bus Creator8/65  "No_filtered_front_left_speed"
  Ground62/1 -> Bus Creator8/85  "GW_EMS_Pot_WhlTrq_Request"
  Ground88/1 -> Bus Creator8/41  "EPS_column_angle"
  Ground16/1 -> Bus Creator8/18  "TCU_ATFailure"
  Ground1/1 -> Bus Creator8/3  "SWS_fault_code"

== system D53_LKAS_JLU_20200909_1512/SignalBusCreator/bsBCMInfo ==
  Bus Creator1 : BusCreator  Inputs=3
  CAN Pack : canmsglib/CAN Pack  CANdbFile=D:\LKAS\Documents\LKAS-Monitor.dbc  MsgList=GW_452_PSA1  MsgName=GW_452_PSA1  MsgIDType=Standard (11-bit identifier)  MsgIdentifier=1106  MsgLength=6  SignalInfo=BCM_Status_Indicator$4$2$2$2$1$0$1$0$-Inf$Inf$#  NSignals=1  StartBits=str2num('[int32(4)]')  SignalSizes=str2num('[int32(2)]')  ByteOrders=str2num('[int32(2)]')  DataTypes=str2num('[int32(2)]')  MultiplexTypes=str2num('[int32(1)]')  MultiplexValues=str2num('[double(0)]')  Factors=str2num('[double(1)]')  Offsets=str2num('[double(0)]')  Minimums=str2num('[double(-Inf)]')  Maximums=str2num('[double(Inf)]')  Remote=off  ApplyMinMax=off  BusOutput=off
      settings: SourceProductName=Simulink Real-Time  SourceProductBaseCode=XP  DataFormat=CANdb specified signals
  CAN Recv (CANRx]) : S-Function  FunctionName=CAN_Rec_P  Parameters=uint8(Module-1),uint32(ID),uint8(Frameformat-1),uint8(Newflag),uint8(FIFO),double(sampletime)  SFunctionDeploymentMode=off  EnableBusSupport=off  mask(CAN_receive){Module=CAN_1, ID=1106, Frameformat=Standard (11-bit identifier), Newflag=off, FIFO=off, sampletime=0.05}
      mask prompts: Module "CAN Port:"; ID "CAN Frame ID:"; Frameformat "CAN Frame Format:"; FIFO "Overflow flag"
      mask init:
      | maskdisplay = canrecicon(Module,ID,Frameformat,Newflag,FIFO);
      | set_param(gcb, 'MaskDisplay', maskdisplay);
      mask TypeOptions Module: CAN_0 | CAN_1 | CAN_2 | CAN_3
      mask TypeOptions Frameformat: Standard (11-bit identifier) | Extended (29-bit identifier)
      mask Display: color('blue');text(0.98,0.9,'MPC5675K','horizontalAlignment','right');color('black');text(0.5,0.6,'FlexCAN_1 Receive','horizontalAlignment','center');text(0.5,0.35,'Standard ID:1106','horizontalAlignment','center');port_label('output',1,'CAN_Msg');
  CAN Send2 : S-Function  FunctionName=CAN_Send_P  Parameters=uint8(CAN_Port-1),uint8(CAN_Priority-1),uint8(S_overflow_flag),uint8(S_timestamp),double(sampletime)  SFunctionDeploymentMode=off  EnableBusSupport=off  mask{CAN_Port=CAN_0, CAN_Priority=3, S_overflow_flag=off, S_timestamp=off, sampletime=0.05}
      mask prompts: CAN_Port "CAN Port:"; CAN_Priority "Priority:"; S_overflow_flag "Send overflow flag"; S_timestamp "Send time stamp"
      mask init:
      | maskdisplay = cansendicon(CAN_Port,CAN_Priority,S_overflow_flag,S_timestamp);
      | set_param(gcb, 'MaskDisplay', maskdisplay);
      mask TypeOptions CAN_Port: CAN_0 | CAN_1 | CAN_2 | CAN_3
      mask TypeOptions CAN_Priority: 0 | 1 | 2 | 3 | 4 | 5 | 6 | 7
      mask Display: color('blue');text(0.98,0.9,'MPC5675K','horizontalAlignment','right');color('black');text(0.5,0.6,'FlexCAN_0 Send','horizontalAlignment','center');text(0.5,0.35,'Priority:3','horizontalAlignment','center');port_label('input',1,'CAN_Msg');
  CAN Unpack : canmsglib/CAN Unpack  CANdbFile=D:\Work\02_LKA\LKAS\Documents\D53-PSA1CAN.dbc  MsgList=GW_452_PSA1  MsgName=GW_452_PSA1  MsgIDType=Standard (11-bit identifier)  MsgIdentifier=1106  MsgLength=6  SignalInfo=BCM_BrakeLampStatus$0$2$2$2$1$0$1$0$0$3$#BCM_CHMSLStatus$2$2$2$2$1$0$1$0$0$3$#BCM_State_Front_Wiper$6$2$2$2$1$0$1$0$-Inf$Inf$#BCM_Status_Indicator$4$2$2$2$1$0$1$0$-Inf$Inf$#Checksum452$40$4$2$2$1$0$1$0$0$15$#GW_BCM_Brakeonly_Request_BCM$18$1$2$2$1$0$1$0$-Inf$Inf$#IC_FCW_Sensitivity$25$2$2$2$1$0$1$0$-Inf$Inf$#IC_Fcw_Activation_Config$20$2$2$2$1$0$1$0$-Inf$Inf$#IC_passengerBeltSwitchSig$19$1$2$2$1$0$1$0$-Inf$Inf$#MP5_AEB_Activation_Config$32$2$2$2$1$0$1$0$-Inf$Inf$#RollingCount_BCM$28$4$2$2$1$0$1$0$0$15$#Speed_Limitation_On$22$1$2$2$1$0$1$0$-Inf$Inf$#TCU_PROGRAMME_ACC$46$2$2$2$1$0$1$0$-Inf$Inf$#  NSignals=13  IDPort=off  TimestampPort=off  ErrorPort=off  RemotePort=off  LengthPort=off  StatusPort=off  StartBits=str2num('[int32(0);int32(2);int32(6);int32(4);int32(40);int32(18);int32(25);int32(20);int32(19);int32(32);int32(28);int32(22);int32(46)]')  SignalSizes=str2num('[int32(2);int32(2);int32(2);int32(2);int32(4);int32(1);int32(2);int32(2);int32(1);int32(2);int32(4);int32(1);int32(2)]')  ByteOrders=str2num('[int32(2);int32(2);int32(2);int32(2);int32(2);int32(2);int32(2);int32(2);int32(2);int32(2);int32(2);int32(2);int32(2)]')  DataTypes=str2num('[int32(2);int32(2);int32(2);int32(2);int32(2);int32(2);int32(2);int32(2);int32(2);int32(2);int32(2);int32(2);int32(2)]')  MultiplexTypes=str2num('[int32(1);int32(1);int32(1);int32(1);int32(1);int32(1);int32(1);int32(1);int32(1);int32(1);int32(1);int32(1);int32(1)]')  MultiplexValues=str2num('[double(0);double(0);double(0);double(0);double(0);double(0);double(0);double(0);double(0);double(0);double(0);double(0);double(0)]')  Factors=str2num('[double(1);double(1);double(1);double(1);double(1);double(1);double(1);double(1);double(1);double(1);double(1);double(1);double(1)]')  Offsets=str2num('[double(0);double(0);double(0);double(0);double(0);double(0);double(0);double(0);double(0);double(0);double(0);double(0);double(0)]')  Minimums=str2num('[double(0);double(0);double(-Inf);double(-Inf);double(0);double(-Inf);double(-Inf);double(-Inf);double(-Inf);double(-Inf);double(0);double(-Inf);double(-Inf)]')  Maximums=str2num('[double(3);double(3);double(Inf);double(Inf);double(15);double(Inf);double(Inf);double(Inf);double(Inf);double(Inf);double(15);double(Inf);double(Inf)]')  ApplyMinMax=off
      settings: SourceProductName=Simulink Real-Time  SourceProductBaseCode=XP  DataFormat=CANdb specified signals
  Data Type Conversion4 : DataTypeConversion  OutDataTypeStr=uint8
  MATLAB Function : MATLAB Function  TreatAsAtomicUnit=on
  Rate Transition3 : RateTransition  OutPortSampleTime=0.01
  Terminator{,1..11} (12 alike) : Terminator
  bsBESState : Outport
  wires:
  CAN Unpack/10 -> Terminator8/1
  CAN Unpack/8 -> Terminator6/1
  Bus Creator1/1 -> bsBESState/1  "bsBESState"
  CAN Unpack/3 -> Terminator2/1
  MATLAB Function/1(Double_Light) -> Bus Creator1/1  "BCM_Double_Light"
  CAN Unpack/11 -> Terminator9/1
  CAN Recv (CANRx])/1 -> CAN Unpack/1
  CAN Unpack/2 -> Terminator1/1
  Data Type Conversion4/1 -> MATLAB Function/1(StLamp)
  CAN Unpack/13 -> Terminator11/1
  CAN Unpack/6 -> Terminator4/1
  CAN Unpack/12 -> Terminator10/1
  CAN Unpack/5 -> Terminator3/1
  CAN Unpack/4 -> CAN Pack/1, Rate Transition3/1
  Rate Transition3/1 -> Data Type Conversion4/1
  CAN Unpack/7 -> Terminator5/1
  MATLAB Function/2(Lft_Light) -> Bus Creator1/2  "BCM_Left_Light"
  MATLAB Function/3(Rgt_light) -> Bus Creator1/3  "BCM_Right_Light"
  CAN Unpack/9 -> Terminator7/1
  CAN Unpack/1 -> Terminator/1
  CAN Pack/1 -> CAN Send2/1

== system D53_LKAS_JLU_20200909_1512/SignalBusCreator/bsEPSInfo ==
  Bus Creator2 : BusCreator  Inputs=9
  CAN Pack : canmsglib/CAN Pack  CANdbFile=D:\LKAS\Documents\LKAS-Monitor.dbc  MsgList=EPS_495_PSA1  MsgName=EPS_495_PSA1  MsgIDType=Standard (11-bit identifier)  MsgIdentifier=1173  MsgLength=4  SignalInfo=State_of_EPS_for_LKA_function$18$3$2$2$1$0$1$0$0$7$#Steering_wheel_torque$0$8$2$1$1$0$2.500000e-01$0$-32$3.150000e+01$#  NSignals=2  StartBits=str2num('[int32(18);int32(0)]')  SignalSizes=str2num('[int32(3);int32(8)]')  ByteOrders=str2num('[int32(2);int32(2)]')  DataTypes=str2num('[int32(2);int32(1)]')  MultiplexTypes=str2num('[int32(1);int32(1)]')  MultiplexValues=str2num('[double(0);double(0)]')  Factors=str2num('[double(1);double(2.500000e-01)]')  Offsets=str2num('[double(0);double(0)]')  Minimums=str2num('[double(0);double(-32)]')  Maximums=str2num('[double(7);double(3.150000e+01)]')  Remote=off  ApplyMinMax=off  BusOutput=off
      settings: SourceProductName=Simulink Real-Time  SourceProductBaseCode=XP  DataFormat=CANdb specified signals
  CAN Recv : S-Function  FunctionName=CAN_Rec_P  Parameters=uint8(Module-1),uint32(ID),uint8(Frameformat-1),uint8(Newflag),uint8(FIFO),double(sampletime)  SFunctionDeploymentMode=off  EnableBusSupport=off  mask(CAN_receive){Module=CAN_1, ID=1173, Frameformat=Standard (11-bit identifier), Newflag=off, FIFO=off, sampletime=0.01}
      mask prompts: Module "CAN Port:"; ID "CAN Frame ID:"; Frameformat "CAN Frame Format:"; FIFO "Overflow flag"
      mask init:
      | maskdisplay = canrecicon(Module,ID,Frameformat,Newflag,FIFO);
      | set_param(gcb, 'MaskDisplay', maskdisplay);
      mask TypeOptions Module: CAN_0 | CAN_1 | CAN_2 | CAN_3
      mask TypeOptions Frameformat: Standard (11-bit identifier) | Extended (29-bit identifier)
      mask Display: color('blue');text(0.98,0.9,'MPC5675K','horizontalAlignment','right');color('black');text(0.5,0.6,'FlexCAN_1 Receive','horizontalAlignment','center');text(0.5,0.35,'Standard ID:1173','horizontalAlignment','center');port_label('output',1,'CAN_Msg');
  CAN Send2 : S-Function  FunctionName=CAN_Send_P  Parameters=uint8(CAN_Port-1),uint8(CAN_Priority-1),uint8(S_overflow_flag),uint8(S_timestamp),double(sampletime)  SFunctionDeploymentMode=off  EnableBusSupport=off  mask{CAN_Port=CAN_0, CAN_Priority=3, S_overflow_flag=off, S_timestamp=off, sampletime=0.01}
      mask prompts: CAN_Port "CAN Port:"; CAN_Priority "Priority:"; S_overflow_flag "Send overflow flag"; S_timestamp "Send time stamp"
      mask init:
      | maskdisplay = cansendicon(CAN_Port,CAN_Priority,S_overflow_flag,S_timestamp);
      | set_param(gcb, 'MaskDisplay', maskdisplay);
      mask TypeOptions CAN_Port: CAN_0 | CAN_1 | CAN_2 | CAN_3
      mask TypeOptions CAN_Priority: 0 | 1 | 2 | 3 | 4 | 5 | 6 | 7
      mask Display: color('blue');text(0.98,0.9,'MPC5675K','horizontalAlignment','right');color('black');text(0.5,0.6,'FlexCAN_0 Send','horizontalAlignment','center');text(0.5,0.35,'Priority:3','horizontalAlignment','center');port_label('input',1,'CAN_Msg');
  CAN Unpack : canmsglib/CAN Unpack  CANdbFile=D:\Work\02_LKA\LKAS\Documents\D53-PSA1CAN.dbc  MsgList=EPS_495_PSA1  MsgName=EPS_495_PSA1  MsgIDType=Standard (11-bit identifier)  MsgIdentifier=1173  MsgLength=4  SignalInfo=Power_steering_status$14$2$2$2$1$0$1$0$-Inf$Inf$#State_indicating_steering_or_not$17$1$2$2$1$0$1$0$-Inf$Inf$#State_of_EPS_for_LKA_function$18$3$2$2$1$0$1$0$-Inf$Inf$#Steering_wheel_torque$0$8$2$1$1$0$2.500000e-01$0$-32$3.150000e+01$#Torque_limitation_if_DAE_limit$16$1$2$2$1$0$1$0$-Inf$Inf$#  NSignals=5  IDPort=off  TimestampPort=off  ErrorPort=off  RemotePort=off  LengthPort=off  StatusPort=off  StartBits=str2num('[int32(14);int32(17);int32(18);int32(0);int32(16)]')  SignalSizes=str2num('[int32(2);int32(1);int32(3);int32(8);int32(1)]')  ByteOrders=str2num('[int32(2);int32(2);int32(2);int32(2);int32(2)]')  DataTypes=str2num('[int32(2);int32(2);int32(2);int32(1);int32(2)]')  MultiplexTypes=str2num('[int32(1);int32(1);int32(1);int32(1);int32(1)]')  MultiplexValues=str2num('[double(0);double(0);double(0);double(0);double(0)]')  Factors=str2num('[double(1);double(1);double(1);double(2.500000e-01);double(1)]')  Offsets=str2num('[double(0);double(0);double(0);double(0);double(0)]')  Minimums=str2num('[double(-Inf);double(-Inf);double(-Inf);double(-32);double(-Inf)]')  Maximums=str2num('[double(Inf);double(Inf);double(Inf);double(3.150000e+01);double(Inf)]')  ApplyMinMax=off
      settings: SourceProductName=Simulink Real-Time  SourceProductBaseCode=XP  DataFormat=CANdb specified signals
  Data Type Conversion : DataTypeConversion  OutDataTypeStr=uint8
  Data Type Conversion1 : DataTypeConversion  OutDataTypeStr=single
  Data Type Conversion2 : DataTypeConversion  OutDataTypeStr=uint8
  Data Type Conversion3 : DataTypeConversion  OutDataTypeStr=uint8
  Ground{,1..4} (5 alike) : Ground
  Rate Transition{1..4} (4 alike) : RateTransition  Deterministic=off  OutPortSampleTime=0.01
  Terminator : Terminator
  bsEPSInfo : Outport
  wires:
  Data Type Conversion/1 -> Bus Creator2/1  "EPS_LKA_State"
  CAN Unpack/3 -> Rate Transition3/1, CAN Pack/1
  Ground/1 -> Bus Creator2/4  "EPS_Trq_State"
  Ground4/1 -> Bus Creator2/8  "EPS_LKA_Current"
  Data Type Conversion2/1 -> Bus Creator2/3  "EPS_Error_State"
  CAN Unpack/1 -> Rate Transition1/1
  CAN Recv/1 -> CAN Unpack/1
  Ground3/1 -> Bus Creator2/7  "EPS_TrqLim_State"
  Data Type Conversion1/1 -> Bus Creator2/2  "EPS_SW_Trq"
  Data Type Conversion3/1 -> Bus Creator2/9  "EPS_SWHold_State"
  CAN Unpack/4 -> CAN Pack/2, Rate Transition4/1
  CAN Unpack/2 -> Rate Transition2/1
  Ground2/1 -> Bus Creator2/6  "SAS_Trim_State"
  CAN Unpack/5 -> Terminator/1
  Ground1/1 -> Bus Creator2/5  "SAS_Clb_State"
  Bus Creator2/1 -> bsEPSInfo/1  "bsEPSInfo"
  Rate Transition1/1 -> Data Type Conversion2/1
  Rate Transition2/1 -> Data Type Conversion3/1
  Rate Transition3/1 -> Data Type Conversion/1
  Rate Transition4/1 -> Data Type Conversion1/1
  CAN Pack/1 -> CAN Send2/1

== system D53_LKAS_JLU_20200909_1512/SignalBusCreator/bsMP5Info ==
  Bus Creator : BusCreator  Inputs=3
  CAN Pack : canmsglib/CAN Pack  CANdbFile=D:\LKAS\Documents\LKAS-Monitor.dbc  MsgList=GW_550_PSA1  MsgName=GW_550_PSA1  MsgIDType=Standard (11-bit identifier)  MsgIdentifier=1360  MsgLength=8  SignalInfo=LC_Mode$6$2$2$2$1$0$1$0$0$3$#LKA_main_switch$5$1$2$2$1$0$1$0$0$1$#  NSignals=2  StartBits=str2num('[int32(6);int32(5)]')  SignalSizes=str2num('[int32(2);int32(1)]')  ByteOrders=str2num('[int32(2);int32(2)]')  DataTypes=str2num('[int32(2);int32(2)]')  MultiplexTypes=str2num('[int32(1);int32(1)]')  MultiplexValues=str2num('[double(0);double(0)]')  Factors=str2num('[double(1);double(1)]')  Offsets=str2num('[double(0);double(0)]')  Minimums=str2num('[double(0);double(0)]')  Maximums=str2num('[double(3);double(1)]')  Remote=off  ApplyMinMax=off  BusOutput=off
      settings: SourceProductName=Simulink Real-Time  SourceProductBaseCode=XP  DataFormat=CANdb specified signals
  CAN Recv : S-Function  FunctionName=CAN_Rec_P  Parameters=uint8(Module-1),uint32(ID),uint8(Frameformat-1),uint8(Newflag),uint8(FIFO),double(sampletime)  SFunctionDeploymentMode=off  EnableBusSupport=off  mask(CAN_receive){Module=CAN_1, ID=1360, Frameformat=Standard (11-bit identifier), Newflag=off, FIFO=off, sampletime=0.5}
      mask prompts: Module "CAN Port:"; ID "CAN Frame ID:"; Frameformat "CAN Frame Format:"; FIFO "Overflow flag"
      mask init:
      | maskdisplay = canrecicon(Module,ID,Frameformat,Newflag,FIFO);
      | set_param(gcb, 'MaskDisplay', maskdisplay);
      mask TypeOptions Module: CAN_0 | CAN_1 | CAN_2 | CAN_3
      mask TypeOptions Frameformat: Standard (11-bit identifier) | Extended (29-bit identifier)
      mask Display: color('blue');text(0.98,0.9,'MPC5675K','horizontalAlignment','right');color('black');text(0.5,0.6,'FlexCAN_1 Receive','horizontalAlignment','center');text(0.5,0.35,'Standard ID:1360','horizontalAlignment','center');port_label('output',1,'CAN_Msg');
  CAN Send2 : S-Function  FunctionName=CAN_Send_P  Parameters=uint8(CAN_Port-1),uint8(CAN_Priority-1),uint8(S_overflow_flag),uint8(S_timestamp),double(sampletime)  SFunctionDeploymentMode=off  EnableBusSupport=off  mask{CAN_Port=CAN_0, CAN_Priority=3, S_overflow_flag=off, S_timestamp=off, sampletime=0.5}
      mask prompts: CAN_Port "CAN Port:"; CAN_Priority "Priority:"; S_overflow_flag "Send overflow flag"; S_timestamp "Send time stamp"
      mask init:
      | maskdisplay = cansendicon(CAN_Port,CAN_Priority,S_overflow_flag,S_timestamp);
      | set_param(gcb, 'MaskDisplay', maskdisplay);
      mask TypeOptions CAN_Port: CAN_0 | CAN_1 | CAN_2 | CAN_3
      mask TypeOptions CAN_Priority: 0 | 1 | 2 | 3 | 4 | 5 | 6 | 7
      mask Display: color('blue');text(0.98,0.9,'MPC5675K','horizontalAlignment','right');color('black');text(0.5,0.6,'FlexCAN_0 Send','horizontalAlignment','center');text(0.5,0.35,'Priority:3','horizontalAlignment','center');port_label('input',1,'CAN_Msg');
  CAN Unpack1 : canmsglib/CAN Unpack  CANdbFile=D:\Work\02_LKA\LKAS\Documents\D53-PSA1CAN.dbc  MsgList=GW_550_PSA1  MsgName=GW_550_PSA1  MsgIDType=Standard (11-bit identifier)  MsgIdentifier=1360  MsgLength=8  SignalInfo=GW_Mp5_ISA_Switch$3$2$2$2$1$0$1$0$0$3$#GW_Mp5_TSR_Switch$1$2$2$2$1$0$1$0$0$3$#LC_Mode$6$2$2$2$1$0$1$0$0$3$#LKA_main_switch$5$1$2$2$1$0$1$0$0$1$#  NSignals=4  IDPort=off  TimestampPort=off  ErrorPort=off  RemotePort=off  LengthPort=off  StatusPort=off  StartBits=str2num('[int32(3);int32(1);int32(6);int32(5)]')  SignalSizes=str2num('[int32(2);int32(2);int32(2);int32(1)]')  ByteOrders=str2num('[int32(2);int32(2);int32(2);int32(2)]')  DataTypes=str2num('[int32(2);int32(2);int32(2);int32(2)]')  MultiplexTypes=str2num('[int32(1);int32(1);int32(1);int32(1)]')  MultiplexValues=str2num('[double(0);double(0);double(0);double(0)]')  Factors=str2num('[double(1);double(1);double(1);double(1)]')  Offsets=str2num('[double(0);double(0);double(0);double(0)]')  Minimums=str2num('[double(0);double(0);double(0);double(0)]')  Maximums=str2num('[double(3);double(3);double(3);double(1)]')  ApplyMinMax=off
      settings: SourceProductName=Simulink Real-Time  SourceProductBaseCode=XP  DataFormat=CANdb specified signals
  Data Type Conversion : DataTypeConversion  OutDataTypeStr=uint8
  Data Type Conversion1 : DataTypeConversion  OutDataTypeStr=uint8
  Ground : Ground
  Rate Transition : RateTransition  Deterministic=off  OutPortSampleTime=0.01
  Rate Transition1 : RateTransition  Deterministic=off  OutPortSampleTime=0.01
  Terminator : Terminator
  Terminator1 : Terminator
  bsMP5Info : Outport
  wires:
  Rate Transition/1 -> Data Type Conversion/1
  CAN Unpack1/2 -> Terminator1/1
  Ground/1 -> Bus Creator/3  "LDW_Warn_Mode"
  CAN Unpack1/1 -> Terminator/1
  Data Type Conversion1/1 -> Bus Creator/1  "LKA_Mode"
  CAN Unpack1/3 -> CAN Pack/1, Rate Transition1/1
  Data Type Conversion/1 -> Bus Creator/2  "LKA_Main_Switch"
  Bus Creator/1 -> bsMP5Info/1  "bsMP5Info"
  CAN Recv/1 -> CAN Unpack1/1
  CAN Unpack1/4 -> CAN Pack/2, Rate Transition/1
  Rate Transition1/1 -> Data Type Conversion1/1
  CAN Pack/1 -> CAN Send2/1
